simulink model "Labda"  (Simulink 7.8)
settings: Solver=ode45  StartTime=0.0  StopTime=inf  RelTol=1e-3
libraries: vrlib x2, simulink x1
settings Model: Creator=valaki  LastModifiedBy=valaki

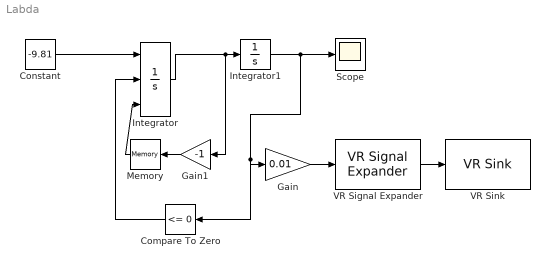
== system Labda ==
  Compare To Zero : simulink/Logic and Bit Operations/Compare To Zero  relop=<=  OutDataTypeStr=boolean
  Constant : Constant  Value=-9.81
  Gain : Gain  Gain=0.01
  Gain1 : Gain  Gain=-1
  Integrator : Integrator  ExternalReset=rising  InitialConditionSource=external
  Integrator1 : Integrator  InitialCondition=2000
  Memory : Memory
  Scope : Scope
  VR Signal Expander : vrlib/VR Signal Expander  outwidth=3  outidx=[2]
  VR Sink : vrlib/VR Sink  SampleTime=0.1  ViewEnable=on  RemoteChange=off  RemoteView=off  FieldsWritten=Ball.translation.3.1.1.double  WorldFileName=C:\Users\valaki\Desktop\labda.wrl  AutoView=off  VideoDimensions=[]  AllowVariableSize=off
  wires:
  Constant/1 -> Integrator/1
  Integrator/1 -> Integrator1/1, Gain1/1
  Integrator1/1 -> Scope/1, Gain/1, Compare To Zero/1
  VR Signal Expander/1 -> VR Sink/1
  Gain/1 -> VR Signal Expander/1
  Compare To Zero/1 -> Integrator/2
  Gain1/1 -> Memory/1
  Memory/1 -> Integrator/3
